simulink model "sanhsovatlyvoinguyentacdautien"  (R2022a)
settings: Solver=VariableStepAuto  StartTime=0.0  StopTime=10.0  RelTol=1e-3
libraries: arduinolib x2
settings Model: Creator=TUAN  LastModifiedBy=TUAN

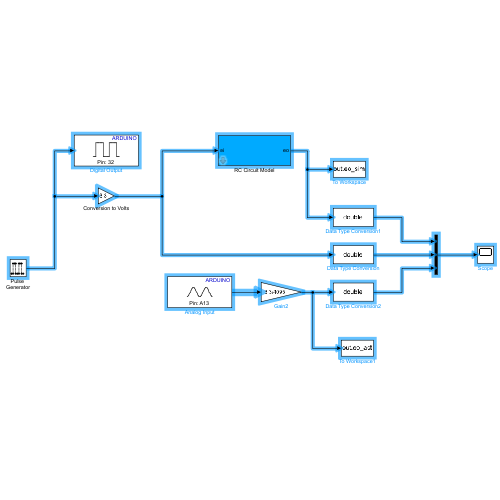
[thumbnail: Simulink's stored preview of the top-level diagram]
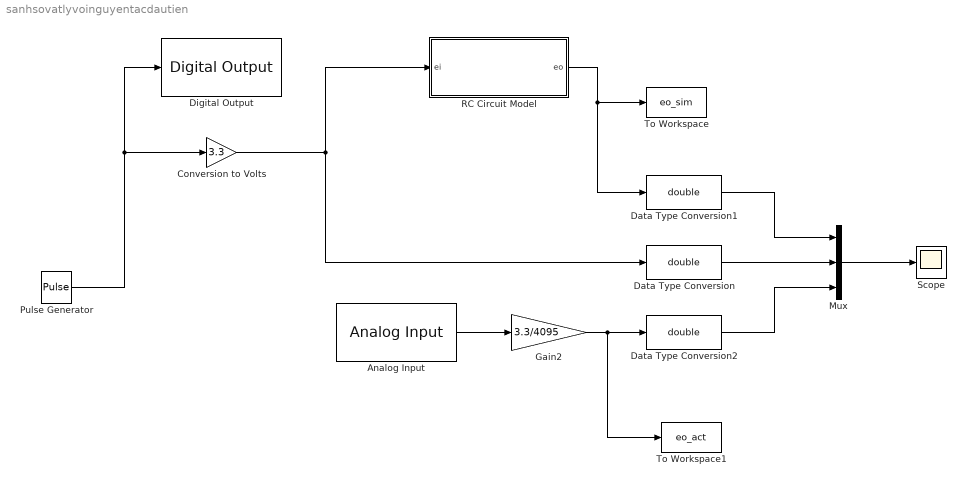
== system sanhsovatlyvoinguyentacdautien ==
  Analog Input : arduinolib/Analog Input  pinNumber=13  ReadResultsOnly=off  ConversionTriggerSource=Software  ExternalTriggerType=uint32( 0 )  OutputDataType=uint16  EnableConversionCompleteNotify=off  EnableOuputStatus=off  SampleTime=-1  blockPlatform=arduino
  Conversion to Volts : Gain  Gain=3.3
  Data Type Conversion : DataTypeConversion  OutDataTypeStr=double  SaturateOnIntegerOverflow=off  RndMeth=Floor
  Data Type Conversion1 : DataTypeConversion  OutDataTypeStr=double  SaturateOnIntegerOverflow=off  RndMeth=Floor
  Data Type Conversion2 : DataTypeConversion  OutDataTypeStr=double  SaturateOnIntegerOverflow=off  RndMeth=Floor
  Digital Output : arduinolib/Digital Output  pinNumber=32  Direction=output  blockPlatform=arduino
  Gain2 : Gain  Gain=3.3/4095
  Mux : Mux  Inputs=3
  Pulse Generator : DiscretePulseGenerator  Period=100  PulseWidth=50  PhaseDelay=50  SampleTime=0.1
  RC Circuit Model : Subsystem  mask{R=10*10^3, C=100*10^-6, q_init=0}
      mask prompts: R "Resistance"; C "Capacitance"; q_init "Initial charge on capacitor"
      mask Display:
      | port_label('input',1,'ei')
      | port_label('output',1,'eo')
  Scope : Scope
  To Workspace : ToWorkspace  VariableName=eo_sim  SampleTime=-1
      settings: Save2DSignal=2-D array (concatenate along first dimension)
  To Workspace1 : ToWorkspace  VariableName=eo_act  SampleTime=-1
      settings: Save2DSignal=2-D array (concatenate along first dimension)
  wires:
  Data Type Conversion2/1 -> Mux/3
  Data Type Conversion1/1 -> Mux/1
  Gain2/1 -> To Workspace1/1, Data Type Conversion2/1
  RC Circuit Model/1(eo) -> To Workspace/1, Data Type Conversion1/1
  Pulse Generator/1 -> Digital Output/1, Conversion to Volts/1
  Mux/1 -> Scope/1
  Data Type Conversion/1 -> Mux/2
  Conversion to Volts/1 -> Data Type Conversion/1, RC Circuit Model/1(ei)
  Analog Input/1 -> Gain2/1

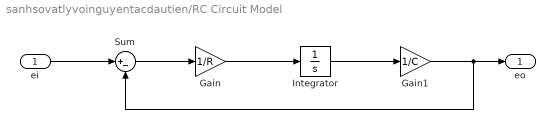
== system sanhsovatlyvoinguyentacdautien/RC Circuit Model ==
  ei : Inport
  Gain : Gain  Gain=1/R
  Gain1 : Gain  Gain=1/C
  Integrator : Integrator  InitialCondition=q_init
  Sum : Sum  Inputs=|+-
  eo : Outport  VectorParamsAs1DForOutWhenUnconnected=off
  wires:
  Integrator/1 -> Gain1/1
  Gain/1 -> Integrator/1
  Gain1/1 -> eo/1, Sum/2
  Sum/1 -> Gain/1
  ei/1 -> Sum/1
